simulink model "L1_5"  (Simulink 7.9)
settings: Solver=ode45  StartTime=0.0  StopTime=8  RelTol=1e-3
libraries: simulink x1
settings Model: Creator=Павло  LastModifiedBy=Павло

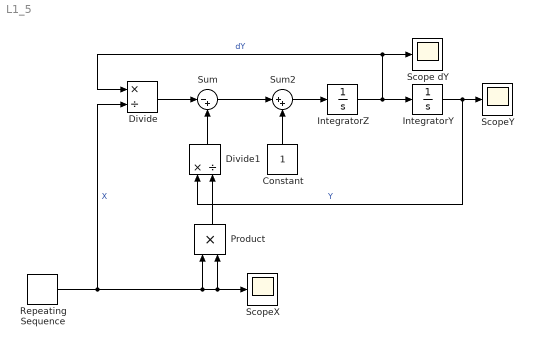
== system L1_5 ==
  Constant : Constant
  Divide : Product  Inputs=*/
  Divide1 : Product  Inputs=*/
  IntegratorY : Integrator  InitialCondition=6
  IntegratorZ : Integrator  InitialCondition=3
  Product : Product  RndMeth=Zero
  Repeating Sequence : simulink/Sources/Repeating Sequence  rep_seq_t=[0 8]  rep_seq_y=[3 11]
  Scope dY : Scope
      settings: TickLabels=on  TimeRange=0.9379378758757522  YMin=0.2922020202020199  YMax=0.54820202020202
  ScopeX : Scope
      settings: TickLabels=on  TimeRange=0.9379378758757522  YMin=0.2922020202020199  YMax=0.54820202020202  SaveName=ScopeData2
  ScopeY : Scope
  Sum : Sum  Inputs=|-+
  Sum2 : Sum  Inputs=|++
  wires:
  IntegratorY/1 -> ScopeY/1, Divide1/1  "Y"
  Repeating Sequence/1 -> Product/2, ScopeX/1, Product/1, Divide/2  "X"
  IntegratorZ/1 -> IntegratorY/1, Scope dY/1, Divide/1  "dY"
  Constant/1 -> Sum2/2
  Sum2/1 -> IntegratorZ/1
  Sum/1 -> Sum2/1
  Divide1/1 -> Sum/2
  Divide/1 -> Sum/1
  Product/1 -> Divide1/2
